simulink model "katayamacopter_ros"  (R2021b)
settings: Solver=VariableStepAuto  StartTime=0.0  StopTime=50  RelTol=1e-3
values from neighbouring files (symbols this model uses):
  duty_b = (u_b - 3.7394) / 0.7158    [calc_inputs.m]
libraries: robotlib x7, mpclib x3
settings Model: VariantFading=off  Creator=marik  LastModifiedBy=amsl
settings DebuggingCC: UnconnectedInputMsg=none  UnconnectedOutputMsg=none  UnconnectedLineMsg=none  UnderSpecifiedDimensionMsg=warning
settings RTWCC: DLArmComputeVersion=20.02.1

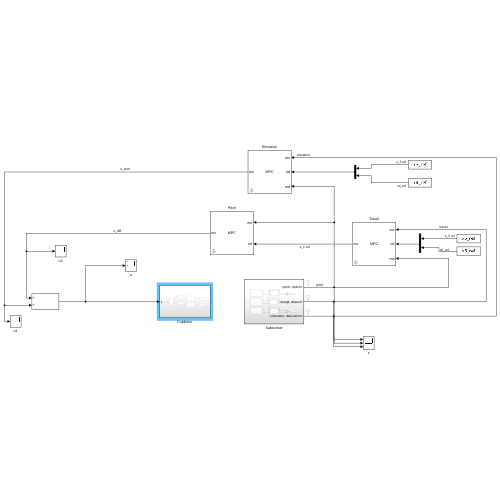
[thumbnail: Simulink's stored preview of the top-level diagram]
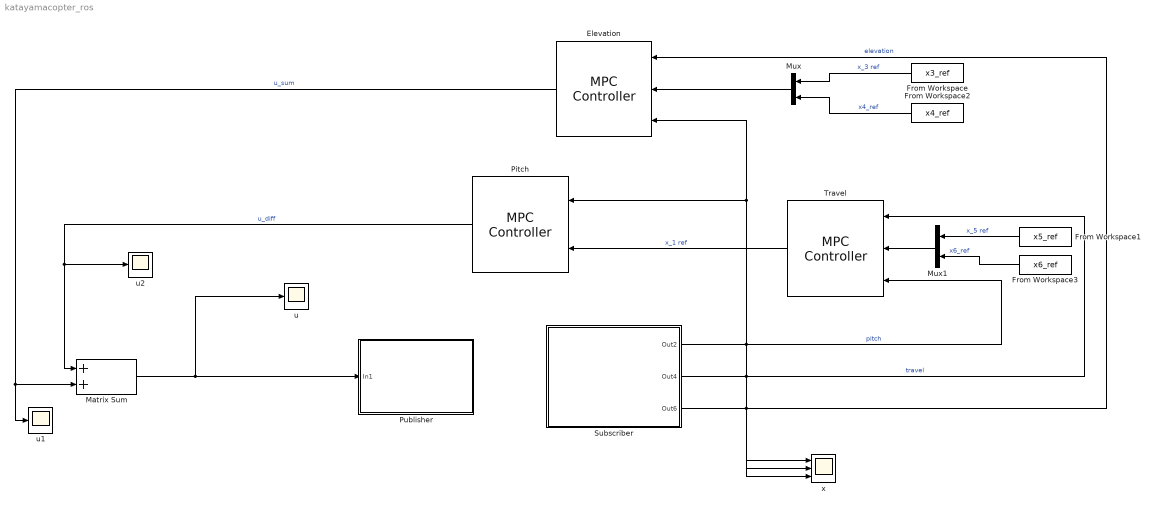
== system katayamacopter_ros ==
  Elevation : mpclib/MPC Controller  SCDEnableBlockLinearizationSpecification=on  mpcobj=mpcelev  is_multiple=0  enable_value=0  return_u0=off  updateMPCinCallerWorkspace=on  md_inport=on  mv_inport=off  uref_inport=off  return_cost=off  return_mvseq=off  return_qpstatus=off  return_xseq=off  return_state=off  return_ovseq=off  state_inport=off  umin_inport=off  umax_inport=off  ymin_inport=off  ymax_inport=off  cc_inport=off  ywt_inport=off  uwt_inport=off  duwt_inport=off  rhoeps_inport=off  pm_inport=off  MaximumP=10  HorizonChoice=FixedHorizon  n_ts=0.02  n_p=15  n_mv=2  n_md=1  n_ud=0  n_mo=2  n_uo=0  BlockDataType=double  SampleTimeInherited=off  switch_inport=off
  From Workspace : FromWorkspace  VariableName=x3_ref  SampleTime=0.1  OutputAfterFinalValue=Holding final value
  From Workspace1 : FromWorkspace  VariableName=x5_ref  SampleTime=0.1  OutputAfterFinalValue=Holding final value
  From Workspace2 : FromWorkspace  VariableName=x4_ref
  From Workspace3 : FromWorkspace  VariableName=x6_ref
  Matrix Sum : Sum
  Mux : Mux  Inputs=2
  Mux1 : Mux  Inputs=2
  Pitch : mpclib/MPC Controller  SCDEnableBlockLinearizationSpecification=on  mpcobj=mpcpitch  is_multiple=0  enable_value=0  return_u0=off  updateMPCinCallerWorkspace=on  md_inport=off  mv_inport=off  uref_inport=off  return_cost=off  return_mvseq=off  return_qpstatus=off  return_xseq=off  return_state=off  return_ovseq=off  state_inport=off  umin_inport=off  umax_inport=off  ymin_inport=off  ymax_inport=off  cc_inport=off  ywt_inport=off  uwt_inport=off  duwt_inport=off  rhoeps_inport=off  pm_inport=off  MaximumP=10  HorizonChoice=FixedHorizon  n_ts=0.008  n_p=80  n_mv=2  n_md=0  n_ud=0  n_mo=2  n_uo=0  BlockDataType=double  SampleTimeInherited=off  switch_inport=off
  Publisher : Subsystem
  Subscriber : Subsystem
  Travel : mpclib/MPC Controller  SCDEnableBlockLinearizationSpecification=on  mpcobj=mpctravel  is_multiple=0  enable_value=0  return_u0=off  updateMPCinCallerWorkspace=on  md_inport=on  mv_inport=off  uref_inport=off  return_cost=off  return_mvseq=off  return_qpstatus=off  return_xseq=off  return_state=off  return_ovseq=off  state_inport=off  umin_inport=off  umax_inport=off  ymin_inport=off  ymax_inport=off  cc_inport=off  ywt_inport=off  uwt_inport=off  duwt_inport=off  rhoeps_inport=off  pm_inport=off  MaximumP=10  HorizonChoice=FixedHorizon  n_ts=0.008  n_p=80  n_mv=2  n_md=1  n_ud=0  n_mo=2  n_uo=0  BlockDataType=double  SampleTimeInherited=off  switch_inport=off
  u : Scope
  u1 : Scope
  u2 : Scope
  x : Scope  NumInputPorts=3
  wires:
  Travel/1 -> Pitch/2  "x_1 ref"
  From Workspace/1 -> Mux/1  "x_3 ref"
  Subscriber/3(Out6) -> x/1, Elevation/1  "elevation"
  Subscriber/1(Out2) -> Elevation/3, Pitch/1, x/2, Travel/3  "pitch"
  Subscriber/2(Out4) -> x/3, Travel/1  "travel"
  From Workspace1/1 -> Mux1/1  "x_5 ref"
  Elevation/1 -> u1/1, Matrix Sum/2  "u_sum"
  Pitch/1 -> u2/1, Matrix Sum/1  "u_diff"
  Matrix Sum/1 -> Publisher/1(In1), u/1
  From Workspace2/1 -> Mux/2  "x4_ref"
  Mux/1 -> Elevation/2
  Mux1/1 -> Travel/2
  From Workspace3/1 -> Mux1/2  "x6_ref"

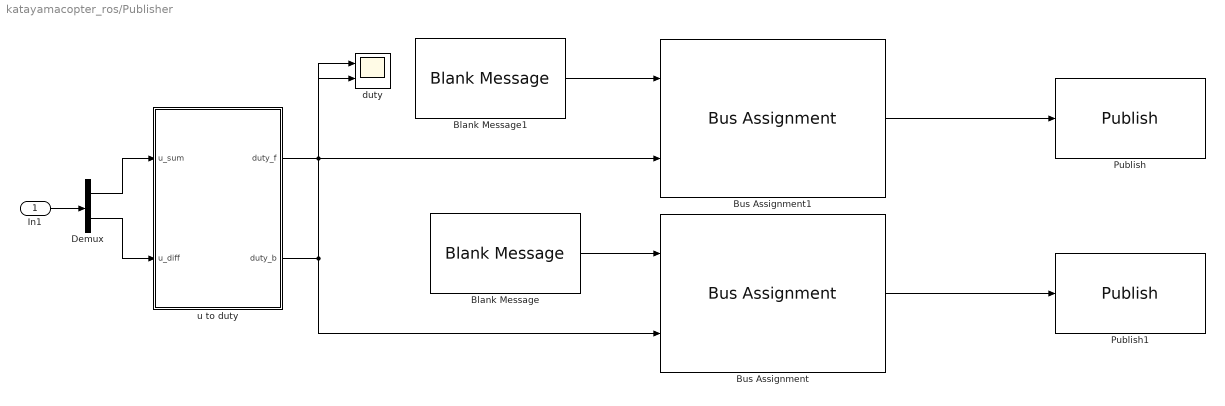
== system katayamacopter_ros/Publisher ==
  In1 : Inport
  Blank Message : robotlib/Blank Message  messageClass=Message  entityType=std_msgs/Float64  messageType=std_msgs/Float64  SampleTime=inf  legacyBusStruct=off
  Blank Message1 : robotlib/Blank Message  messageClass=Message  entityType=std_msgs/Float64  messageType=std_msgs/Float64  SampleTime=inf  legacyBusStruct=off
  Bus Assignment : BusAssignment  AssignedSignals=Data
  Bus Assignment1 : BusAssignment  AssignedSignals=Data
  Demux : Demux  Outputs=2
  Publish : robotlib/Publish  topicSource=Specify your own  topic=/duty_b  messageType=std_msgs/Float64  legacyBusStruct=off  messageQueueLength=1
  Publish1 : robotlib/Publish  topicSource=Specify your own  topic=/duty_a  messageType=std_msgs/Float64  legacyBusStruct=off  messageQueueLength=1
  duty : Scope  NumInputPorts=2
  u to duty : MATLAB Function  TreatAsAtomicUnit=on
  wires:
  Demux/2 -> u to duty/2(u_diff)
  u to duty/1(duty_f) -> duty/1, Bus Assignment1/2
  u to duty/2(duty_b) -> Bus Assignment/2, duty/2
  In1/1 -> Demux/1
  Demux/1 -> u to duty/1(u_sum)
  Blank Message/1 -> Bus Assignment/1
  Bus Assignment/1 -> Publish1/1
  Blank Message1/1 -> Bus Assignment1/1
  Bus Assignment1/1 -> Publish/1

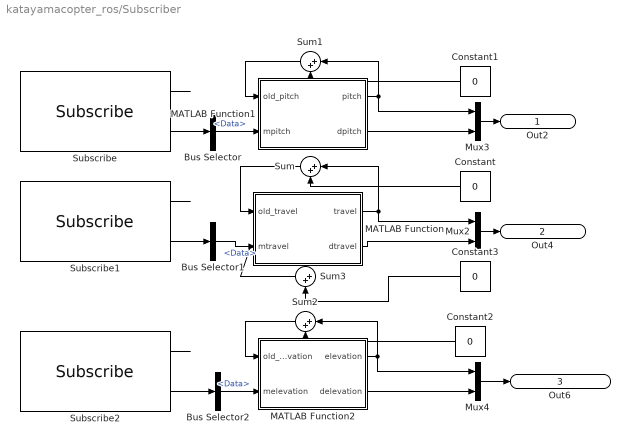
== system katayamacopter_ros/Subscriber ==
  Bus Selector : BusSelector  OutputSignals=Data
  Bus Selector1 : BusSelector  OutputSignals=Data
  Bus Selector2 : BusSelector  OutputSignals=Data
  Constant{,1..3} (4 alike) : Constant  Value=0
  MATLAB Function : MATLAB Function  TreatAsAtomicUnit=on
  MATLAB Function1 : MATLAB Function  TreatAsAtomicUnit=on
  MATLAB Function2 : MATLAB Function  TreatAsAtomicUnit=on
  Mux2 : Mux  Inputs=2
  Mux3 : Mux  Inputs=2
  Mux4 : Mux  Inputs=2
  Subscribe : robotlib/Subscribe  topicSource=Specify your own  topic=/pitch  messageType=std_msgs/Float64  SampleTime=-1  legacyBusStruct=off  messageQueueLength=1
  Subscribe1 : robotlib/Subscribe  topicSource=Specify your own  topic=/travel  messageType=std_msgs/Float64  SampleTime=-1  legacyBusStruct=off  messageQueueLength=1
  Subscribe2 : robotlib/Subscribe  topicSource=Specify your own  topic=/elevation  messageType=std_msgs/Float64  SampleTime=-1  legacyBusStruct=off  messageQueueLength=1
  Sum{,1..3} (4 alike) : Sum  Inputs=|++
  Out2 : Outport
  Out4 : Outport  Port=2
  Out6 : Outport  Port=3
  wires:
  Subscribe2/2 -> Bus Selector2/1
  MATLAB Function/2(dtravel) -> Mux2/2
  Subscribe1/2 -> Bus Selector1/1
  MATLAB Function1/2(dpitch) -> Mux3/2
  Subscribe/2 -> Bus Selector/1
  Mux2/1 -> Out4/1
  MATLAB Function1/1(pitch) -> Sum1/1, Mux3/1
  Subscribe2/1 -> ?
  Mux3/1 -> Out2/1
  Mux4/1 -> Out6/1
  Subscribe1/1 -> ?
  Subscribe/1 -> ?
  MATLAB Function/1(travel) -> Sum/1, Mux2/1
  MATLAB Function2/2(delevation) -> Mux4/2
  MATLAB Function2/1(elevation) -> Sum2/1, Mux4/1
  Bus Selector/1 -> MATLAB Function1/2(mpitch)  "<Data>"
  Bus Selector1/1 -> MATLAB Function/2(mtravel)  "<Data>"
  Bus Selector2/1 -> MATLAB Function2/2(melevation)  "<Data>"
  Sum/1 -> MATLAB Function/1(old_travel)
  Constant/1 -> Sum/2
  Constant1/1 -> Sum1/2
  Sum1/1 -> MATLAB Function1/1(old_pitch)
  Constant2/1 -> Sum2/2
  Sum2/1 -> MATLAB Function2/1(old_elevation)
  Constant3/1 -> Sum3/2
  ? -> Sum3/1
  Sum3/1 -> ?

== matlab function katayamacopter_ros/Subscriber/MATLAB Function ==
  data: old_travel input; mtravel input; travel output; dtravel output
function [travel,dtravel] = fcn(old_travel,mtravel)
hz = 10;
travel = mtravel;
if travel == 0
    old_travel = 0;
end
dtravel = (mtravel - old_travel) * hz;

== matlab function katayamacopter_ros/Publisher/u to duty ==
  data: u_sum input; duty_f output; u_diff input; duty_b output
function [duty_f , duty_b] = fcn(u_sum,u_diff)
%sum/diff to forword/back
% u_sum = u_f + u_b
% u_diff = u_f - u_b
% ∴
% u_f = (u_sum + u_diff) / 2
% u_b = (u_sum - u_diff) / 2

u_f = (u_sum + u_diff) / 2;
u_b = (u_sum - u_diff) / 2;

%%
%u to duty
% 数値は片山の卒論fig4.3
duty_f = (u_f + 3.3235) / 0.6386 /100 * 0.95;
duty_b = (u_b + 3.7394) / 0.7158 /100 * 0.9;

== matlab function katayamacopter_ros/Subscriber/MATLAB Function1 ==
  data: old_pitch input; mpitch input; pitch output; dpitch output
function [pitch,dpitch] = fcn(old_pitch,mpitch)
hz = 10;
%pitch = mpitch.data;
pitch = mpitch * pi / 180;
if pitch == 0
    old_pitch = 0;
end
dpitch = (pitch - old_pitch) * hz;

== matlab function katayamacopter_ros/Subscriber/MATLAB Function2 ==
  data: old_elevation input; melevation input; elevation output; delevation output
function [elevation,delevation] = fcn(old_elevation,melevation)
hz = 10;
%elevation = melevation.data;
elevation = melevation * pi / 180;
if elevation == 0
    old_elevation = 0;
end
delevation = (elevation - old_elevation) * hz;
